simulink model "exp5_4"  (Simulink 7.7)
settings: Solver=VariableStepDiscrete  SolverMode=SingleTasking  StartTime=0.0  StopTime=10.0  RelTol=1e-3  AbsTol=1e-6
settings Model: Creator=Administrator  LastModifiedBy=Administrator  ExtModeTrigMode=oneshot  ExtModeArmWhenConnect=off
settings DataIOCC: LimitDataPoints=off
settings OptimizationCC: BlockReduction=off  BooleanDataType=off
settings DebuggingCC: SaveWithParameterizedLinksMsg=none  SignalResolutionControl=TryResolveAllWithWarning  SolverPrmCheckMsg=none  MultiTaskDSMMsg=warning  MultiTaskCondExecSysMsg=none  StrictBusMsg=None
settings HardwareCC: TargetUnknown=on
settings RTWCC: TemplateMakefile=grt_vc.tmf  IncludeERTFirstTime=on

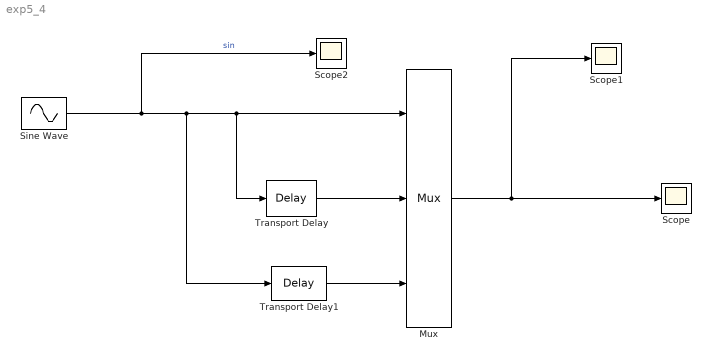
== system exp5_4 ==
  Mux : Mux  Inputs=3
  Scope : Scope
      settings: TickLabels=on  TimeRange=10  YMin=-2  YMax=2  DataFormat=Array
  Scope1 : Scope
      settings: TickLabels=on  TimeRange=10  YMin=-2  YMax=2  DataFormat=Array
  Scope2 : Scope
      settings: TickLabels=on  TimeRange=10  YMin=-2  YMax=2  DataFormat=Array
  Sine Wave : Sin  SampleTime=0
  Transport Delay : TransportDelay
  Transport Delay1 : TransportDelay  DelayTime=2
  wires:
  Transport Delay/1 -> Mux/2
  Transport Delay1/1 -> Mux/3
  Sine Wave/1 -> Transport Delay1/1, Mux/1, Transport Delay/1, Scope2/1  "sin"
  Mux/1 -> Scope1/1, Scope/1
